simulink model "GHV_open_toolbox"  (R2023b)
settings: Solver=VariableStepAuto  StartTime=0.0  StopTime=10  FixedStep=0.0000001  MaxStep=0.001  RelTol=1e-3
InitFcn:
  | run('init.m')
values from neighbouring files (symbols this model uses):
  GHV_cfg = struct()    [GHV_Configuration.m]
libraries: aerolibasang x3, simulink_extras x2, shared6dof x1, aerolibadyn x1, aerolibatmos2 x1
settings Model: SimulationMode=accelerator  Creator=Admin  LastModifiedBy=Admin
settings SolverCC: AllowMultiTaskInputOutput=on  ZeroCrossControl=EnableAll  ZeroCrossAlgorithm=Adaptive  AutoInsertRateTranBlk=on

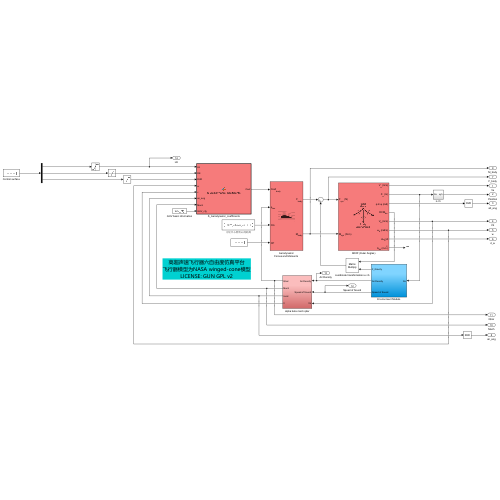
[thumbnail: Simulink's stored preview of the top-level diagram]
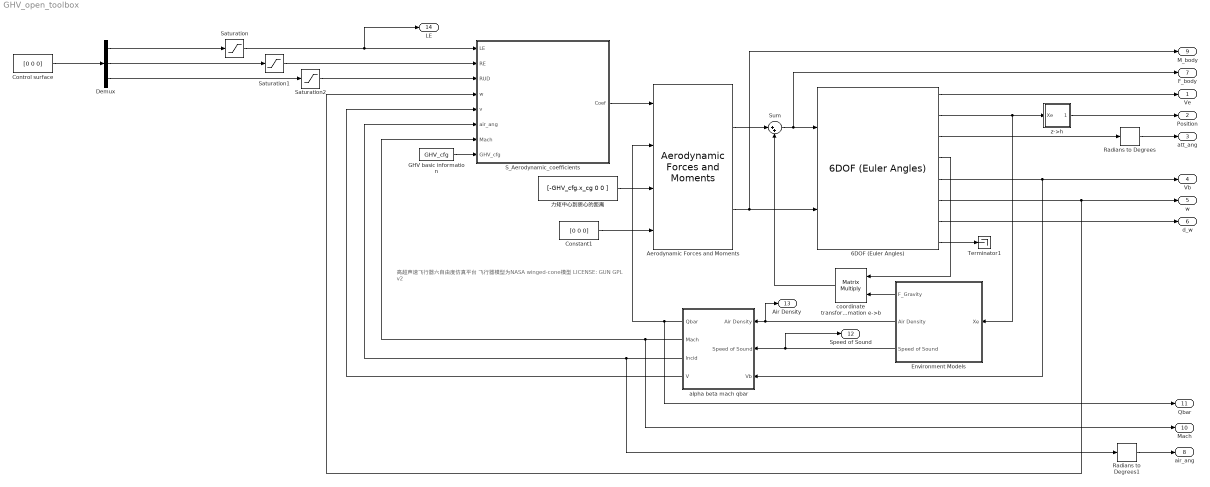
== system GHV_open_toolbox ==
  note: 高超声速飞行器六自由度仿真平台
      | 飞行器模型为NASA winged-cone模型
      | LICENSE: GUN GPL v2
  6DOF (Euler Angles) : shared6dof/6DOF (Euler Angles)  units=Metric (MKS)  mtype=Fixed  rep=Euler Angles  xme_0=Position_init  Vm_0=Speed_init  eul_0=Euler_init  pm_0=Omega_init  mass_0=GHV_cfg.mass_full  mass_e=0.5  mass_f=2.0  inertia=GHV_cfg.J  inertia_e=eye(3)  inertia_f=2*eye(3)  k_quat=1.0  vre_flag=on  abi_flag=off  aMode=0  xme_statename=''  Vm_statename=''  eul_statename=''  quat_statename=''  pm_statename=''  mass_statename=''
  "Aerodynamic Forces and Moments " : aerolibadyn/Aerodynamic Forces and Moments   inputAxes=Body  outputForceAxes=Body  outputMomentAxes=Body  S=GHV_cfg.s_ref  b=GHV_cfg.b_ref  cbar=GHV_cfg.c_ref
  Constant1 : Constant  Value=[0 0 0]
  Control surface : Constant  Value=[0 0 0]
  Demux : Demux  Outputs=3
  Environment Models : Subsystem
  GHV basic information : Constant  Value=GHV_cfg  VectorParams1D=off  OutDataTypeStr=Bus: slBus1
  Radians to Degrees : simulink_extras/Transformations/Radians to Degrees
  Radians to Degrees1 : simulink_extras/Transformations/Radians to Degrees
  S_Aerodynamic_coefficients : MATLAB Function  TreatAsAtomicUnit=on
  Saturation : Saturate  UpperLimit=30  LowerLimit=-30
  Saturation1 : Saturate  UpperLimit=30  LowerLimit=-30
  Saturation2 : Saturate  UpperLimit=30  LowerLimit=-30
  Sum : Sum  Inputs=|++
  Terminator1 : Terminator
  alpha beta mach qbar : Subsystem
  coordinate transformation e->b : Product  Multiplication=Matrix(*)
  z->h : Subsystem
  力矩中心到质心的距离 : Constant  Value=[-GHV_cfg.x_cg 0 0 ]
  Ve : Outport
  Position : Outport  Port=2
  att_ang : Outport  Port=3
  Vb : Outport  Port=4
  w : Outport  Port=5
  d_w : Outport  Port=6
  F_body : Outport  Port=7
  air_ang : Outport  Port=8
  M_body : Outport  Port=9
  Mach : Outport  Port=10
  Qbar : Outport  Port=11
  Speed of Sound : Outport  Port=12
  Air Density : Outport  Port=13
  LE : Outport  Port=14
  wires:
  "Aerodynamic Forces and Moments "/1 -> Sum/1
  "Aerodynamic Forces and Moments "/2 -> M_body/1, 6DOF (Euler Angles)/2
  S_Aerodynamic_coefficients/1(Coef) -> "Aerodynamic Forces and Moments "/1
  Environment Models/1(F_Gravity) -> coordinate transformation e->b/2
  6DOF (Euler Angles)/4 -> coordinate transformation e->b/1
  Sum/1 -> F_body/1, 6DOF (Euler Angles)/1
  coordinate transformation e->b/1 -> Sum/2
  6DOF (Euler Angles)/2 -> z->h/1(Xe), Environment Models/1(Xe)
  Environment Models/3(Speed of Sound) -> Speed of Sound/1, alpha beta mach qbar/2(Speed of Sound)
  Environment Models/2(Air Density) -> Air Density/1, alpha beta mach qbar/1(Air Density)
  6DOF (Euler Angles)/5 -> Vb/1, alpha beta mach qbar/3(Vb)
  alpha beta mach qbar/1(Qbar) -> Qbar/1, "Aerodynamic Forces and Moments "/2
  alpha beta mach qbar/3(Incid) -> Radians to Degrees1/1, S_Aerodynamic_coefficients/6(air_ang)
  alpha beta mach qbar/4(V) -> S_Aerodynamic_coefficients/5(v)
  alpha beta mach qbar/2(Mach) -> Mach/1, S_Aerodynamic_coefficients/7(Mach)
  力矩中心到质心的距离/1 -> "Aerodynamic Forces and Moments "/3
  Constant1/1 -> "Aerodynamic Forces and Moments "/4
  6DOF (Euler Angles)/1 -> Ve/1
  6DOF (Euler Angles)/3 -> Radians to Degrees/1
  6DOF (Euler Angles)/7 -> d_w/1
  6DOF (Euler Angles)/8 -> Terminator1/1
  Control surface/1 -> Demux/1
  GHV basic information/1 -> S_Aerodynamic_coefficients/8(GHV_cfg)
  z->h/1(xyh) -> Position/1
  Radians to Degrees/1 -> att_ang/1
  Radians to Degrees1/1 -> air_ang/1
  Demux/1 -> Saturation/1
  Demux/2 -> Saturation1/1
  Demux/3 -> Saturation2/1
  6DOF (Euler Angles)/6 -> S_Aerodynamic_coefficients/4(w), w/1
  Saturation/1 -> LE/1, S_Aerodynamic_coefficients/1(LE)
  Saturation1/1 -> S_Aerodynamic_coefficients/2(RE)
  Saturation2/1 -> S_Aerodynamic_coefficients/3(RUD)

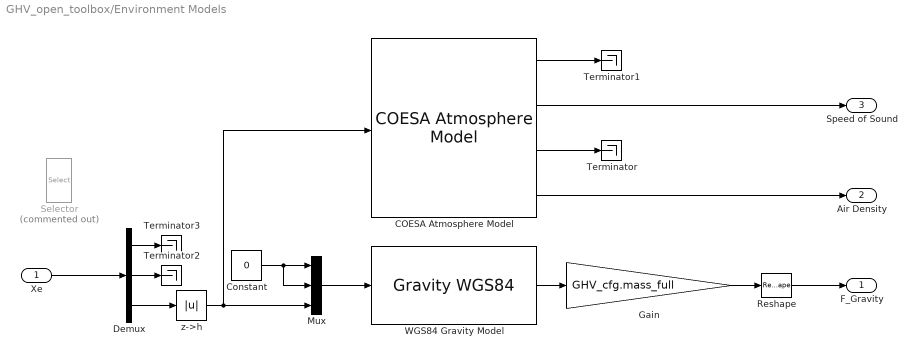
== system GHV_open_toolbox/Environment Models ==
  Xe : Inport
  COESA Atmosphere Model : aerolibatmos2/COESA Atmosphere Model  units=Metric (MKS)  spec=1976 COESA-extended U.S. Standard Atmosphere  model=Profile  profile_var=High temperature  profile_percent=1%  profile_alt=5 km (16404 ft)  envelope_var=High temperature  envelope_percent=1%  action=Warning
  Constant : Constant  Value=0
  Demux : Demux  Outputs=3
  Gain : Gain  Gain=GHV_cfg.mass_full
  Mux : Mux  Inputs=3
  Reshape : Reshape
  Selector : Selector  Commented=on  InputPortWidth=3  IndexOptions=Index vector (dialog)  Indices=[3]  OutputSizes=1
  Terminator{,1..3} (4 alike) : Terminator
  "WGS84 Gravity Model  " : GravityWGS84  action=None
  z->h : Abs  SaturateOnIntegerOverflow=off
  F_Gravity : Outport
  Air Density : Outport  Port=2
  Speed of Sound : Outport  Port=3
  wires:
  Gain/1 -> Reshape/1
  Constant/1 -> Mux/2, Mux/1
  z->h/1 -> COESA Atmosphere Model/1, Mux/3
  Mux/1 -> "WGS84 Gravity Model  "/1
  COESA Atmosphere Model/1 -> Terminator1/1
  COESA Atmosphere Model/2 -> Speed of Sound/1
  COESA Atmosphere Model/3 -> Terminator/1
  "WGS84 Gravity Model  "/1 -> Gain/1
  COESA Atmosphere Model/4 -> Air Density/1
  Reshape/1 -> F_Gravity/1
  Xe/1 -> Demux/1
  Demux/3 -> z->h/1
  Demux/2 -> Terminator2/1
  Demux/1 -> Terminator3/1

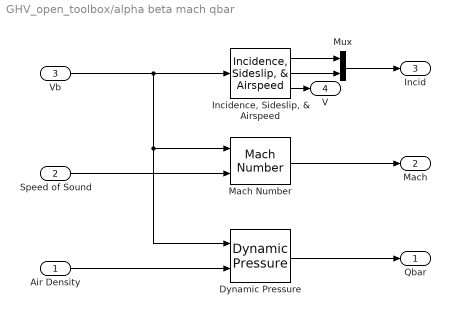
== system GHV_open_toolbox/alpha beta mach qbar ==
  Air Density : Inport
  Speed of Sound : Inport  Port=2
  Vb : Inport  Port=3
  Dynamic Pressure : aerolibasang/Dynamic Pressure
  "Incidence, Sideslip, & Airspeed" : aerolibasang/Incidence, Sideslip, & Airspeed
  Mach Number : aerolibasang/Mach Number
  Mux : Mux  Inputs=2
  Qbar : Outport
  Mach : Outport  Port=2
  Incid : Outport  Port=3
  V : Outport  Port=4
  wires:
  Speed of Sound/1 -> Mach Number/2
  Mach Number/1 -> Mach/1
  "Incidence, Sideslip, & Airspeed"/2 -> Mux/2
  Vb/1 -> Dynamic Pressure/1, Mach Number/1, "Incidence, Sideslip, & Airspeed"/1
  Dynamic Pressure/1 -> Qbar/1
  Mux/1 -> Incid/1
  "Incidence, Sideslip, & Airspeed"/1 -> Mux/1
  Air Density/1 -> Dynamic Pressure/2
  "Incidence, Sideslip, & Airspeed"/3 -> V/1

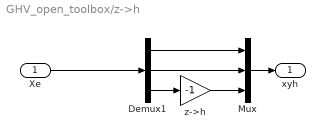
== system GHV_open_toolbox/z->h ==
  Xe : Inport
  Demux1 : Demux  Outputs=3
  Mux : Mux  Inputs=3
  z->h : Gain  Gain=-1
  xyh : Outport
  wires:
  z->h/1 -> Mux/3
  Demux1/2 -> Mux/2
  Demux1/3 -> z->h/1
  Demux1/1 -> Mux/1
  Xe/1 -> Demux1/1
  Mux/1 -> xyh/1

== matlab function GHV_open_toolbox/S_Aerodynamic_coefficients ==
  data: LE input; Coef output; RE input; RUD input; w input; v input; air_ang input; Mach input; GHV_cfg input
function Coef = S_Aerodynamic_coefficients(LE, RE, RUD, w, v, air_ang, Mach, GHV_cfg)
    Coef = zeros(1, 6);
    Coef = Aerodynamic_coefficients(LE, RE, RUD, air_ang, v, w, Mach, GHV_cfg);

end
